simulink model "project3"  (R2023b)
settings: Solver=VariableStepAuto  StartTime=0.0  StopTime=10.0  RelTol=1e-3
libraries: simulink x1
settings Model: Creator=mfb36  LastModifiedBy=mfb36

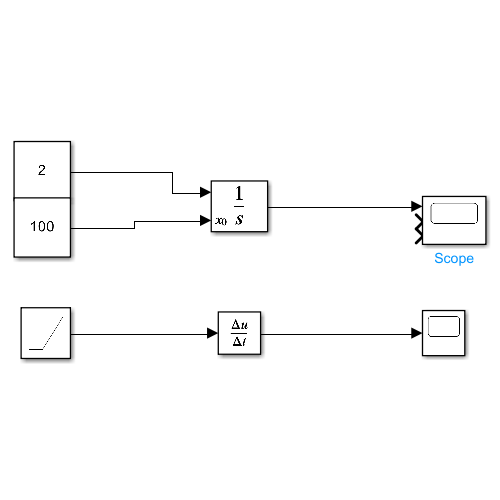
[thumbnail: Simulink's stored preview of the top-level diagram]
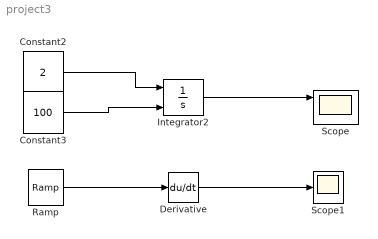
== system project3 ==
  Constant2 : Constant  Value=2
  Constant3 : Constant  Value=100
  Derivative : Derivative
  Integrator2 : Integrator  InitialConditionSource=external
  Ramp : simulink/Sources/Ramp  slope=1  start=0  InitialOutput=0
  Scope : Scope  NumInputPorts=3
  Scope1 : Scope
  wires:
  Derivative/1 -> Scope1/1
  Ramp/1 -> Derivative/1
  Constant2/1 -> Integrator2/1
  Integrator2/1 -> Scope/1
  Constant3/1 -> Integrator2/2
